simulink model "GraphicalFunction3"  (R2020b)
settings: Solver=FixedStepDiscrete  StartTime=0.0  StopTime=0.1  FixedStep=0.1  RelTol=1e-3  EnableMultiTasking=on
settings Model: Creator=bzhan  LastModifiedBy=apple
settings SolverCC: AutoInsertRateTranBlk=on
settings DataIOCC: LimitDataPoints=on
settings OptimizationCC: LifeSpan=inf
settings DebuggingCC: AllowSymbolicDim=off  SFUnexpectedBacktrackingDiag=warning  SFNoUnconditionalDefaultTransitionDiag=warning  SFExecutionAtInitializationDiag=none  ArithmeticOperatorsInVariantConditions=warning
settings SFSimCC: SimUseLocalCustomCode=off  CustomCodeUndefinedFunction=UseInterfaceOnly
settings RTWCC: RTWUseLocalCustomCode=off
settings CodeAppCC: StateflowObjectComments=on
settings GRTTargetCC: TargetLangStandard=C89/C90 (ANSI)
settings ConfigComp: CovMetricSettings=dw  CovSaveCumulativeToWorkspaceVar=on  CovSaveSingleToWorkspaceVar=on  CovExternalEMLEnable=off  CovSFcnEnable=off

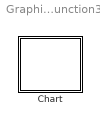
== system GraphicalFunction3 ==
  Chart : Stateflow chart  TreatAsAtomicUnit=on

== stateflow chart GraphicalFunction3/Chart ==
  state index=find(N) [function]
    (junction 2) -> (junction 12) [order 3] : {index=i;}
    (default) -> (junction 2) : {i=1;a=1;}
    (junction 2) -> (junction 10) [order 2] : [i>N]
    (junction 10) -> (junction 12) : {index=-1;}
    (junction 2) -> (junction 5) [order 1] : [i<=N&&a<=2]
    (junction 6) -> (junction 2)
    (junction 5) -> (junction 6) : {i=i+1;a=a+1;}
  state [r,s]=square(i1,j1) [function]
    (default) -> (junction 30)
    (junction 30) -> (junction 33) : {r=i1*i1;}
    (junction 33) -> (junction 34) : {s=j1*j1;}
  state B
    en: f("en_B");
    [x,y]=square(x,y);
    fprintf("%f",x);
    fprintf("%f", x)
  state A
    en: f("en_A")
  (default) -> A
  A -> B : [find(4)==3]
  data: index function_output; N function_input; i1 function_input; j1 function_input; r function_output; s function_output; s function_input; i local; x local double =2; y local double =3
  function f(s):
    | function f(s)
    |   fprintf(s+"\n");
